simulink model "exp9_4"  (R2020a)
settings: Solver=VariableStepAuto  StartTime=0.0  StopTime=10.0  RelTol=1e-3
libraries: simulink x1
settings Model: Creator=zengw  LastModifiedBy=zengw

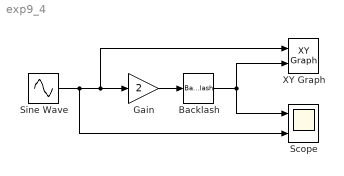
== system exp9_4 ==
  Backlash : Backlash  BacklashWidth=1.6
  Gain : Gain  Gain=2
  Scope : Scope  NumInputPorts=2
  Sine Wave : Sin  Amplitude=5  SampleTime=0
  XY Graph : simulink/Sinks/XY Graph  xmin=-5  xmax=5  ymin=-10  ymax=10  st=-1
  wires:
  Sine Wave/1 -> Gain/1, XY Graph/1, Scope/2
  Backlash/1 -> Scope/1, XY Graph/2
  Gain/1 -> Backlash/1
